simulink model "k6jca_181230_ARDUINO"  (R2018b)
settings: Solver=ode45  StartTime=0.0  StopTime=9000  MaxStep=1  RelTol=1e-3  EnableMultiTasking=on
InitFcn:
  | D=30
settings Model: Creator=Dick  LastModifiedBy=Jeff
settings DataIOCC: LimitDataPoints=on  SaveFormat=Array  SaveOutput=off  SignalLogging=off  DSMLogging=off  SaveTime=off
settings OptimizationCC: LifeSpan=inf
settings DebuggingCC: SFUnexpectedBacktrackingDiag=warning  SFNoUnconditionalDefaultTransitionDiag=warning  SFExecutionAtInitializationDiag=none
settings HardwareCC: ProdBitPerPointer=32  ProdBitPerSizeT=32  ProdBitPerPtrDiffT=32  ProdLargestAtomicFloat=None  ProdIntDivRoundTo=Undefined  ProdEndianess=Unspecified  ProdWordSize=32  ProdHWDeviceType=32-bit Generic
settings ModelReferenceCC: PropagateSignalLabelsOutOfModel=off
settings SFSimCC: SimUseLocalCustomCode=off
settings RTWCC: RTWUseLocalCustomCode=off
settings CodeAppCC: StateflowObjectComments=on
settings GRTTargetCC: TargetLangStandard=C89/C90 (ANSI)  GeneratePreprocessorConditionals=Disable all
settings ConfigComp: CovMetricSettings=dw  CovHtmlReporting=on  CovSaveCumulativeToWorkspaceVar=on  CovSaveSingleToWorkspaceVar=on  CovExternalEMLEnable=off

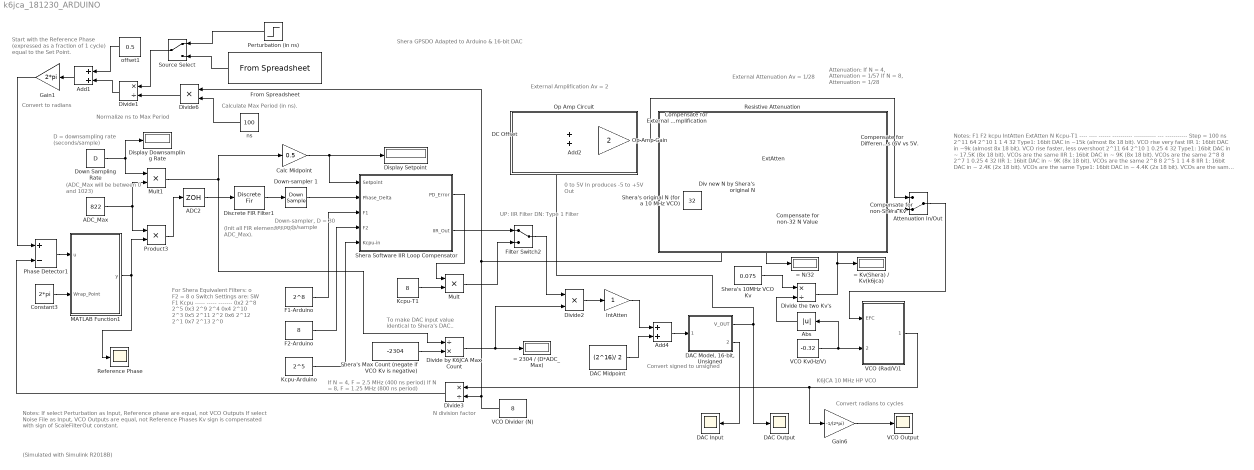
== system k6jca_181230_ARDUINO ==
  note: (Simulated with Simulink R2018B)
  note: Convert
      | signed
      | to unsigned
  note: Attenuation:
      | If N = 4, Attenuation = 1/57
      | If N = 8, Attenuation = 1/28
  note: To make DAC input value
      | identical to Shera's DAC..
  note: Notes:
      | If select Perturbation as Input, Reference phase are equal, not VCO Outputs
      | If select Noise File as Input, VCO Outputs are equal, not Reference Phases
      | Kv sign is compensated with sign of ScaleFilterOut constant.
  note: Normalize ns to
      | Max Period
  note: Calculate Max Period
      | (in ns).
  note: Convert to radians
  note: N division factor
  note: 0 to 5V In produces
      |  -5 to +5V Out
  note: External Attenuation
      | Av = 1/28
  note: D = downsampling rate
      |      (seconds/sample)
  note: If N = 4, F = 2.5 MHz   (400 ns period)
      | If N = 8, F = 1.25 MHz (800 ns period)
  note: (Init all FIR
      | elements to
      | 1/2 ADC_Max).
  note: (ADC_Max will be between 0 and 1023)
  note: Convert radians to cycles
  note: K6JCA 10 MHz HP VCO
  note: UP:  IIR Filter
      | DN:  Type 1 Filter
  note: Shera GPSDO Adapted
      | to Arduino & 16-bit DAC
  note: Start with the Reference Phase
      | (expressed as a fraction of 1 cycle)
      | equal to the Set Point.
  note: External Amplification
      | Av = 2
  note: Down-sampler,
      | D = 30
      | seconds/sample
  note: For Shera Equivalent Filters:
      |      o  F2 = 8
      |      o  Switch Settings are:
      |
      |    SW      F1         Kcpu
      |    -----     -----       -------
      |    0x2     2^8          2^5
      |    0x3     2^9          2^4
      |    0x4     2^10        2^3
      |    0x5     2^11        2^2
      |    0x6     2^12        2^1
      |    0x7     2^13        2^0
  note: Notes:
      | F1 F2 kcpu IntAtten ExtAtten N Kcpu-T1
      | ---- ---- ------ ---------- ----------- --- -----------
      | Step = 100 ns
      | 2^11 64 2^10 1 1 4 32 Type1: 16bit DAC in ~15k (almost 8x 18 bit). VCO rise very fast
      | IIR 1: 16bit DAC in ~9k (almost 8x 18 bit). VCO rise faster, less overshoot
      | 2^11 64 2^10 1 0.25 4 32 Type1: 16bit DAC in ~ 17.5K (8x 18 bit). VCOs are the same
      | IIR 1: 16bit DAC in ~ 9K (8x 18 bit). VCOs are the same
      | 2^8 8 2^7 1 0.25 4 32 IIR 1: 16bit DAC in ~ 9K (8x 18 bit). VCOs are the same
      | 2^8 8 2^5 1 1 4 8 IIR 1: 16bit DAC in ~ 2.4K (2x 18 bit). VCOs are the same
      | Type1: 16bit DAC in ~ 4.4K (2x 18 bit). VCOs are the sam
      |
      | Step = 200 ns
      | 2^8 8 2^5 1 1 4 8 IIR 1: 16bit DAC in ~ 5K (2x 18 bit). VCOs are the same
      |
      | 2^11 64 2^10 1 0.25 8 32 16 bit DAC in = 4x 18 bit (too much if type 1 filter). VCO Outs Equal
      | 2^11 64 2^10 0.25 1 8 32 DAC Inputs equal.. VCO Outs Equal
      | >2^11 64 2^8 1 1 8 8 DAC Inputs equal. VCO Outs Equal
      | >2^8 8 2^5 1 1 8 8 DAC Inputs equal. VCO Outs Equal
      |
      | 2^8 8 2^5 1 1 16 8 IIR1: DAC In = 1.2K (1/2x 18bit). VCO Outs Equal
      | 2^8 8 2^6 1 0.5 16 8 IIR1: DAC Ins equal. VCO Outs Equal
      |
      | Changing IIR Response:
      | 2^8 8 2^7 1 1 4 -- IIR Faster rise, less overshoot, DAC ~ 18K
      | 2^8 8 2^6 1 1 4 -- IIR a bit slower, but still faster, less overshoot, DAC ~ 9K
      | 2^8 8 2^7 1 0.5 4 -- IIR a bit slower, but still faster, less overshoot, DAC ~ 18K
      |
      | 2^8 16 2^5 1 1 4 -- VCO: Lots of ringing
      | 2^8 4 2^5 1 1 4 -- DAC In 9K (almost 4x 16 bit). Less overshoot. Not bad.
      |
      | Note: This last has a nice IIR response, but note that Type 1 filter's rise time is lengthened by 2 due to
      | OtherComp going from 0.5 to 0.25.
      | If try to compensate by increasing it from 16 to 32, DAC input is > 32K.
      |
      | Use:
      | 2^8 8 2^5 1 1 8 8 DAC Inputs equal. VCO Outs Equal
      | 2^8 8 2^5 1 1 4 8 DAC In 2x Shera. VCO Outs Equal
      |
      | To make the DAC inputs w.r.t. DAC full scale comparable:
      | 2^8 8 2^3 1 4 8 2 DAC In =0.25 x Shera. VCO Outs Equal
  = 2304 / (D*ADC_Max) : Display
  = Kv(Shera) / Kv(k6jca) : Display
  = N/32 : Display
  ADC2 : ZeroOrderHold
  ADC_Max : Constant  Value=822  SampleTime=Inf
  Abs : Abs
  Add1 : Sum
  Add2 : Sum
  Add4 : Sum
  Attenuation In/Out : ManualSwitch  CurrentSetting=0
  Calc Midpoint : Gain  Gain=0.5
  "Compensate for non-32 N Value " : Product  Inputs=**
  Compensate for non-Shera Kv : Product  Inputs=**
  Compensate for Different DAC ranges (6V vs 5V. : Gain  Gain=6/5
  Compensate for External Amplification : Gain  Gain=0.5
  Constant3 : Constant  Value=2*pi
  DAC Input : Scope
  DAC Midpoint : Constant  Value=(2^16)/ 2  SampleTime=Inf
  "DAC Model, 16-bit, Unsigned" : Subsystem
  DAC Output : Scope
  DC Offset : Constant  Value=-2.5  SampleTime=Inf
  Discrete FIR Filter1 : DiscreteFir  Coefficients=[1 1 1 1 1 1 1 1 1 1 1 1 1 1 1 1 1 1 1 1 1 1 1 1 1 1 1 1 1 1]  InitialStates=411
  "Display Downsampling Rate " : Display
  Display Setpoint : Display
  "Div new N by Shera's original N " : Product  Inputs=/*
  Divide by K6JCA Max Count : Product  Inputs=/*
  Divide the two Kv's : Product  Inputs=*/
  Divide1 : Product  Inputs=*/
  Divide2 : Product  Inputs=**
  Divide3 : Product  Inputs=*/
  Divide6 : Product  Inputs=**
  "Down Sampling Rate " : Constant  Value=D  SampleTime=D
  Down-sampler 1 : DownSample  N=D  RateOptions=Allow multirate processing
  ExtAtten : Gain
  F1-Arduino : Constant  Value=2^8  SampleTime=Inf
  F2-Arduino : Constant  Value=8  SampleTime=Inf
  Filter Switch2 : ManualSwitch
  From Spreadsheet : FromSpreadsheet  FileName=Trimble_PD_181227.xlsx  SheetName=Sheet3
  Gain1 : Gain  Gain=2*pi
  Gain6 : Gain  Gain=-1/(2*pi)
  IntAtten : Gain
  Kcpu-Arduino : Constant  Value=2^5  SampleTime=Inf
  Kcpu-T1 : Constant  Value=8  SampleTime=Inf
  MATLAB Function1 : MATLAB Function  TreatAsAtomicUnit=on
  Mult : Product  Inputs=**
  Mult1 : Product  Inputs=**
  Op Amp Circuit : Subsystem
      mask Display: disp('')
  Op Amp Gain : Gain  Gain=2
  Perturbation (in ns) : Step  Time=100  After=400  SampleTime=1
  Phase Detector1 : Sum  Inputs=+-
  Product3 : Product
  Reference Phase : Scope
  Resistive Attenuation : Subsystem
      mask Display: disp('')
  Shera Software IIR Loop Compensator : Subsystem
  Shera's original N (for a 10 MHz VCO) : Constant  Value=32  SampleTime=Inf
  Shera's 10MHz VCO Kv : Constant  Value=0.075  SampleTime=Inf
  Shera's Max Count (negate if VCO Kv is negative) : Constant  Value=-2304  SampleTime=Inf
  Source Select : ManualSwitch
  VCO (Rad/V)1 : Subsystem
  VCO Divider (N) : Constant  Value=8  SampleTime=Inf
  VCO Kv(Hz/V) : Constant  Value=-0.32  SampleTime=Inf
  VCO Output : Scope
  ns : Constant  Value=100  SampleTime=Inf
  offset1 : Constant  Value=0.5  VectorParams1D=off  SampleTime=Inf
  wires:
  VCO (Rad/V)1/1(Radians) -> Divide3/1, Gain6/1
  "Compensate for non-32 N Value "/1 -> Compensate for non-Shera Kv/1
  Down-sampler 1/1 -> Shera Software IIR Loop Compensator/2(Phase_Delta)
  offset1/1 -> Add1/1
  Filter Switch2/1 -> Divide2/1
  Gain1/1 -> Phase Detector1/1
  ADC_Max/1 -> Mult1/2, Product3/1
  Shera's original N (for a 10 MHz VCO)/1 -> "Div new N by Shera's original N "/1
  Add2/1 -> Op Amp Gain/1
  Phase Detector1/1 -> MATLAB Function1/1(u)
  F1-Arduino/1 -> Shera Software IIR Loop Compensator/3(F1)
  Kcpu-Arduino/1 -> Shera Software IIR Loop Compensator/5(Kcpu-in)
  DC Offset/1 -> Add2/1
  Compensate for External Amplification/1 -> ExtAtten/1
  "Div new N by Shera's original N "/1 -> "Compensate for non-32 N Value "/2, = N/32/1
  Shera Software IIR Loop Compensator/2("IIR_Out ") -> Filter Switch2/1
  Product3/1 -> ADC2/1
  Shera Software IIR Loop Compensator/1("PD_Error ") -> Mult/1
  Kcpu-T1/1 -> Mult/2
  VCO Kv(Hz/V)/1 -> Abs/1, VCO (Rad/V)1/2(Kv_(Hz/V))
  ADC2/1 -> Discrete FIR Filter1/1
  Divide3/1 -> Phase Detector1/2
  Constant3/1 -> MATLAB Function1/2(Wrap_Point)
  Mult/1 -> Filter Switch2/2
  Compensate for Different DAC ranges (6V vs 5V./1 -> "Compensate for non-32 N Value "/1
  "Down Sampling Rate "/1 -> "Display Downsampling Rate "/1, Mult1/1
  VCO Divider (N)/1 -> Divide3/2, "Div new N by Shera's original N "/2, Divide6/1
  F2-Arduino/1 -> Shera Software IIR Loop Compensator/4(F2)
  ExtAtten/1 -> Compensate for Different DAC ranges (6V vs 5V./1
  Discrete FIR Filter1/1 -> Down-sampler 1/1
  Add1/1 -> Gain1/1
  MATLAB Function1/1(y) -> Reference Phase/1, Product3/2
  "DAC Model, 16-bit, Unsigned"/1(V_OUT) -> DAC Output/1, Add2/2
  Divide1/1 -> Add1/2
  From Spreadsheet/1 -> Source Select/2
  Divide6/1 -> Divide1/2
  ns/1 -> Divide6/2
  Source Select/1 -> Divide1/1
  Perturbation (in ns)/1 -> Source Select/1
  Divide the two Kv's/1 -> Compensate for non-Shera Kv/2, = Kv(Shera) / Kv(k6jca)/1
  Abs/1 -> Divide the two Kv's/2
  Divide2/1 -> IntAtten/1
  Op Amp Gain/1 -> Attenuation In/Out/1, Compensate for External Amplification/1
  Attenuation In/Out/1 -> VCO (Rad/V)1/1(EFC)
  Compensate for non-Shera Kv/1 -> Attenuation In/Out/2
  Add4/1 -> "DAC Model, 16-bit, Unsigned"/1(COUNT_IN)
  IntAtten/1 -> Add4/1
  DAC Midpoint/1 -> Add4/2
  Calc Midpoint/1 -> Shera Software IIR Loop Compensator/1(Setpoint), Display Setpoint/1
  Mult1/1 -> Calc Midpoint/1, Divide by K6JCA Max Count/1
  Shera's Max Count (negate if VCO Kv is negative)/1 -> Divide by K6JCA Max Count/2
  Divide by K6JCA Max Count/1 -> Divide2/2, = 2304 / (D*ADC_Max)/1
  Gain6/1 -> VCO Output/1
  "DAC Model, 16-bit, Unsigned"/2(Quant_OUT1) -> DAC Input/1
  Shera's 10MHz VCO Kv/1 -> Divide the two Kv's/1

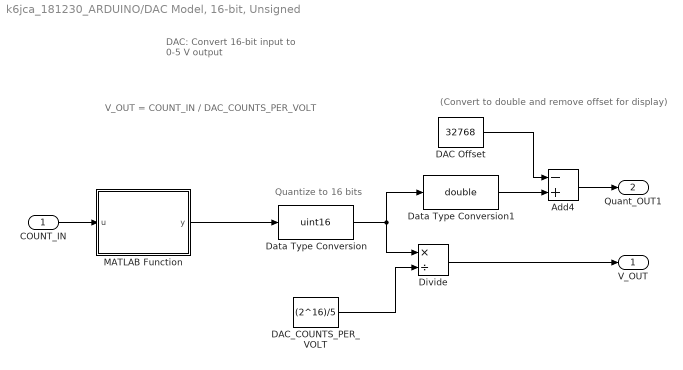
== system k6jca_181230_ARDUINO/DAC Model, 16-bit, Unsigned ==
  note: (Convert to double and remove offset for display)
  note: Quantize to 16 bits
  note: V_OUT = COUNT_IN / DAC_COUNTS_PER_VOLT
  note: DAC:
      | Convert 16-bit input
      | to
      | 0-5 V output
  COUNT_IN : Inport
  Add4 : Sum  Inputs=-+
  DAC Offset : Constant  Value=32768  SampleTime=Inf
  "DAC_COUNTS_PER_VOLT " : Constant  Value=(2^16)/5  SampleTime=Inf
  Data Type Conversion : DataTypeConversion  OutDataTypeStr=uint16
  Data Type Conversion1 : DataTypeConversion  OutDataTypeStr=double
  Divide : Product  Inputs=*/
  MATLAB Function : MATLAB Function  TreatAsAtomicUnit=on
  V_OUT : Outport
  Quant_OUT1 : Outport  Port=2
  wires:
  "DAC_COUNTS_PER_VOLT "/1 -> Divide/2
  Divide/1 -> V_OUT/1
  COUNT_IN/1 -> MATLAB Function/1(u)
  MATLAB Function/1(y) -> Data Type Conversion/1
  Data Type Conversion/1 -> Divide/1, Data Type Conversion1/1
  Add4/1 -> Quant_OUT1/1
  Data Type Conversion1/1 -> Add4/2
  DAC Offset/1 -> Add4/1

== system k6jca_181230_ARDUINO/Op Amp Circuit ==

== system k6jca_181230_ARDUINO/Resistive Attenuation ==

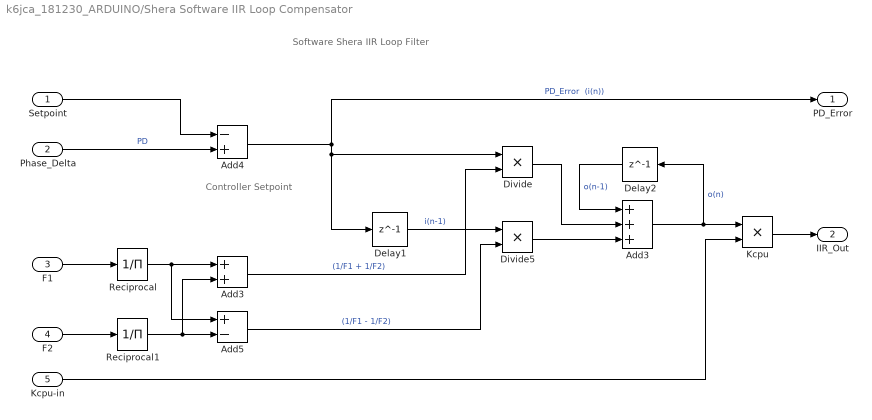
== system k6jca_181230_ARDUINO/Shera Software IIR Loop Compensator ==
  note: Software Shera IIR Loop Filter
  note: Controller
      | Setpoint
  Setpoint : Inport
  Phase_Delta : Inport  Port=2
  F1 : Inport  Port=3
  F2 : Inport  Port=4
  Kcpu-in : Inport  Port=5
  Add3 : Sum
  "Add3 " : Sum  Inputs=+++
  Add4 : Sum  Inputs=-+
  Add5 : Sum  Inputs=+-
  Delay1 : Delay  DelayLength=1
  Delay2 : Delay  DelayLength=1
  Divide : Product  Inputs=**
  Divide5 : Product  Inputs=**
  Kcpu : Product  Inputs=**
  Reciprocal : Product  Inputs=/
  Reciprocal1 : Product  Inputs=/
  "PD_Error " : Outport
  "IIR_Out " : Outport  Port=2
  wires:
  Setpoint/1 -> Add4/1
  Add4/1 -> Divide/1, Delay1/1, "PD_Error "/1  "PD_Error  (i(n))"
  "Add3 "/1 -> Delay2/1, Kcpu/1  "o(n)"
  F1/1 -> Reciprocal/1
  F2/1 -> Reciprocal1/1
  Reciprocal/1 -> Add5/1, Add3/1
  Reciprocal1/1 -> Add5/2, Add3/2
  Add3/1 -> Divide/2  "(1/F1 + 1/F2)"
  Delay1/1 -> Divide5/1  "i(n-1)"
  Add5/1 -> Divide5/2  "(1/F1 - 1/F2)"
  Delay2/1 -> "Add3 "/1  "o(n-1)"
  Divide/1 -> "Add3 "/2
  Divide5/1 -> "Add3 "/3
  Phase_Delta/1 -> Add4/2  "PD"
  Kcpu-in/1 -> Kcpu/2
  Kcpu/1 -> "IIR_Out "/1

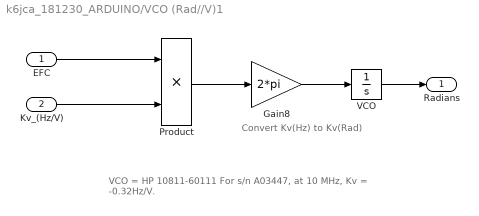
== system k6jca_181230_ARDUINO/VCO (Rad//V)1 ==
  note: VCO = HP 10811-60111
      |
      | For s/n A03447, at 10 MHz, Kv = -0.32Hz/V.
  note: Convert Kv(Hz)
      | to Kv(Rad)
  EFC : Inport
  Kv_(Hz/V) : Inport  Port=2
  Gain8 : Gain  Gain=2*pi
  Product : Product
  VCO : Integrator
  Radians : Outport
  wires:
  Gain8/1 -> VCO/1
  EFC/1 -> Product/1
  Product/1 -> Gain8/1
  VCO/1 -> Radians/1
  Kv_(Hz/V)/1 -> Product/2

== matlab function k6jca_181230_ARDUINO/MATLAB Function1 ==
  data: u input; y output; Wrap_Point input
function y = phase_wrapper(u,Wrap_Point)
%#codegen
y=0;
if u > 0
   y = mod(u,Wrap_Point);
elseif u < 0
   y = Wrap_Point-(mod(-u,Wrap_Point));  
end
y = y/Wrap_Point;  % normalize y to 1.

== matlab function k6jca_181230_ARDUINO/DAC Model, 16-bit, Unsigned/MATLAB Function ==
  data: y output; u input
function y = b16_dac_limiter(u)
%#codegen
% This limits the DAC input to 65535 and 0
%
y = u;
if u > 65535
   y = 65535;
elseif u < 0
   y = 0;  
end
